simulink model "lab_1_position_loop_step"  (R2016a)
settings: Solver=ode3  SolverMode=SingleTasking  StartTime=0.0  StopTime=10  FixedStep=0.01  RelTol=1e-3
undefined symbols (not defined in the file or in its folder): DiscIntNeverNeededParam
libraries: arduinolib x4, simulink x1, neural x1
settings Model: ExtModeTrigDuration=2  Creator=ismail  LastModifiedBy=MSI
settings DataIOCC: LimitDataPoints=on  SaveFormat=Array
settings OptimizationCC: ExpressionDepthLimit=2147483647  OptimizeModelRefInitCode=on  LifeSpan=1  MaxStackSize=64
settings DebuggingCC: UnderspecifiedInitializationDetection=Classic  MergeDetectMultiDrivingBlocksExec=none  StateNameClashWarn=warning
settings HardwareCC: ProdBitPerInt=16  ProdBitPerPointer=16  ProdLargestAtomicFloat=None  ProdWordSize=8  ProdHWDeviceType=Atmel->AVR
settings ModelReferenceCC: PropagateSignalLabelsOutOfModel=off
settings RTWCC: SystemTargetFile=ert.tlc  HardwareBoard=Arduino Uno  TLCOptions=-aInlineSetEventsForThisBaseRateFcn=TLC_FALSE -aSuppressMultiTaskScheduler=TLC_FALSE -aRateBasedStepFcn=1  TemplateMakefile=ert_default_tmf  GenerateReport=on  RTWVerbose=off  Toolchain=Arduino AVR  BuildConfiguration=Faster Runs  IncludeHyperlinkInReport=on  LaunchReport=on  GenerateTraceInfo=on  GenerateTraceReport=on  GenerateTraceReportSl=on  GenerateTraceReportSf=on  GenerateTraceReportEml=on
settings CodeAppCC: ForceParamTrailComments=on  IgnoreCustomStorageClasses=off  OperatorAnnotations=on  SimulinkDataObjDesc=on  SFDataObjDesc=on  MATLABFcnDesc=on  CustomSymbolStrType=$N$R$M  InsertBlockDesc=on  MATLABSourceComments=on  InternalIdentifier=Classic
settings ERTTargetCC: SupportContinuousTime=on  SupportVariableSizeSignals=on

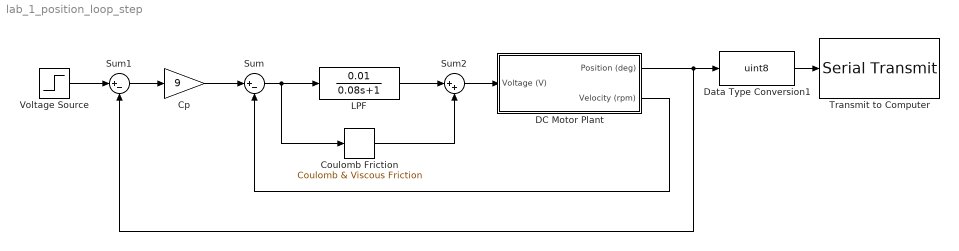
== system lab_1_position_loop_step ==
  Coulomb Friction : simulink/Discontinuities/Coulomb & Viscous Friction  offset=2  gain=0
  Cp : Gain  Gain=9
  DC Motor Plant : Subsystem
  Data Type Conversion1 : DataTypeConversion  OutDataTypeStr=uint8  RndMeth=Round
  LPF : TransferFcn  Numerator=[0.01]  Denominator=[0.08 1]
  Sum : Sum  Inputs=|+-
  Sum1 : Sum  Inputs=|+-
  Sum2 : Sum  Inputs=|++
  Transmit to Computer : arduinolib/Serial Transmit  portNumber=0  sendmode=write  sendformat=Decimal  floatprecision=2  blockPlatform=arduino
  Voltage Source : Step  Time=0  SampleTime=0
  wires:
  DC Motor Plant/1(Position (deg)) -> Sum1/2, Data Type Conversion1/1
  Data Type Conversion1/1 -> Transmit to Computer/1
  Sum/1 -> LPF/1, Coulomb Friction/1
  Cp/1 -> Sum/1
  Sum2/1 -> DC Motor Plant/1(Voltage (V))
  DC Motor Plant/2(Velocity (rpm)) -> Sum/2
  Sum1/1 -> Cp/1
  Voltage Source/1 -> Sum1/1
  LPF/1 -> Sum2/1
  Coulomb Friction/1 -> Sum2/2

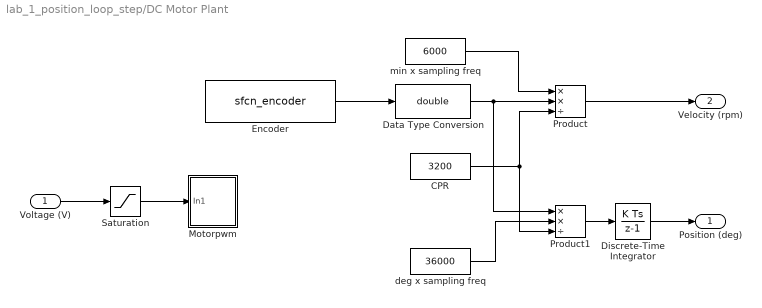
== system lab_1_position_loop_step/DC Motor Plant ==
  Voltage (V) : Inport
  CPR : Constant  Value=3200
  Data Type Conversion : DataTypeConversion  OutDataTypeStr=double  RndMeth=Round
  Discrete-Time Integrator : DiscreteIntegrator  InitialConditionSetting=State (most efficient)  SampleTime=-1  ICPrevOutput=DiscIntNeverNeededParam  ICPrevScaledInput=DiscIntNeverNeededParam
  Encoder : S-Function  InitFcn=try, set_param(gcb,'FunctionName','sfcn_encoder'), end  FunctionName=sfcn_encoder  Parameters=uint8(0),uint8(2),uint8(3)  SFunctionModules=sfcn_encoder_wrapper  SFunctionDeploymentMode=off  EnableBusSupport=off  mask(S-Function Builder){}
      mask init:
      | val = [[.9  0.75 0.75 1 1 .9 .9 1]',[1 1 0.75 0.75 .9 .9 1 .9]'];try , sys = get_param(gcb,'SfunBuilderFcnName');if isempty(sys), sys = get_param(gcb,'FunctionName'); end,catch, sys = get_param(gcb,'FunctionName'); end
      settings: CopyFcn=set_param(gcbh,'LinkStatus','none')  PreSaveFcn=try, set_param(gcb,'FunctionName','sfcn_encoder'), end  OpenFcn=sfunctionwizard(gcbh)
      mask Display: plot(val(:,1),val(:,2)),disp(sys), port_label('output',1,'pos')
  Motorpwm : Subsystem
  Product : Product  Inputs=**/
  Product1 : Product  Inputs=**/
  Saturation : Saturate  UpperLimit=12  LowerLimit=-12
  deg x sampling freq : Constant  Value=36000
  min x sampling freq : Constant  Value=6000
  Position (deg) : Outport
  Velocity (rpm) : Outport  Port=2
  wires:
  Encoder/1 -> Data Type Conversion/1
  Voltage (V)/1 -> Saturation/1
  Data Type Conversion/1 -> Product1/1, Product/2
  Product/1 -> Velocity (rpm)/1
  min x sampling freq/1 -> Product/1
  Product1/1 -> Discrete-Time Integrator/1
  deg x sampling freq/1 -> Product1/2
  Discrete-Time Integrator/1 -> Position (deg)/1
  CPR/1 -> Product1/3, Product/3
  Saturation/1 -> Motorpwm/1(In1)

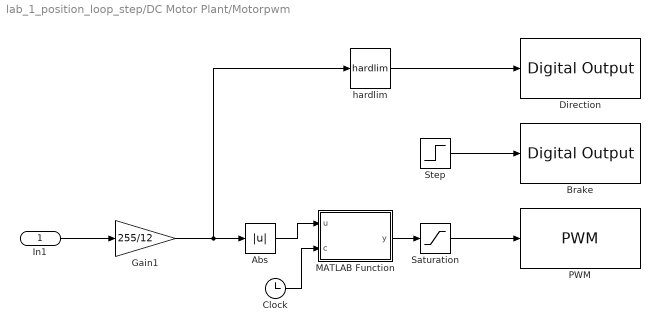
== system lab_1_position_loop_step/DC Motor Plant/Motorpwm ==
  In1 : Inport
  Abs : Abs
  Brake : arduinolib/Digital Output  pinNumber=8  blockPlatform=arduino
  Clock : Clock
  "Direction " : arduinolib/Digital Output  pinNumber=13  blockPlatform=arduino
  Gain1 : Gain  Gain=255/12
  MATLAB Function : MATLAB Function  TreatAsAtomicUnit=on
  PWM : arduinolib/PWM  pinNumber=11  EnableInputFrequency=off  InitialFrequency=2000  InitialDutyCycle=0  NotificationType=None  blockPlatform=arduino
  Saturation : Saturate  UpperLimit=255  LowerLimit=0
  Step : Step  Time=0  After=0  SampleTime=0
  hardlim : neural/Transfer Functions/hardlim
  wires:
  hardlim/1 -> "Direction "/1
  Step/1 -> Brake/1
  Saturation/1 -> PWM/1
  In1/1 -> Gain1/1
  MATLAB Function/1(y) -> Saturation/1
  Abs/1 -> MATLAB Function/1(u)
  Clock/1 -> MATLAB Function/2(c)
  Gain1/1 -> hardlim/1, Abs/1

== matlab function lab_1_position_loop_step/DC Motor Plant/Motorpwm/MATLAB Function ==
  data: u input; y output; c input
function y = fcn(u,c)
%#codegen
if c<10
    y = u;
else
    y=0;
end
